simulink model "Model_Predictive_Controller"  (R2018a)
settings: Solver=VariableStepAuto  StartTime=0.0  StopTime=10.0  RelTol=1e-3
libraries: Meldas_library x2, mpclib x1
settings Model: Creator=KAARTIK  LastModifiedBy=KAARTIK

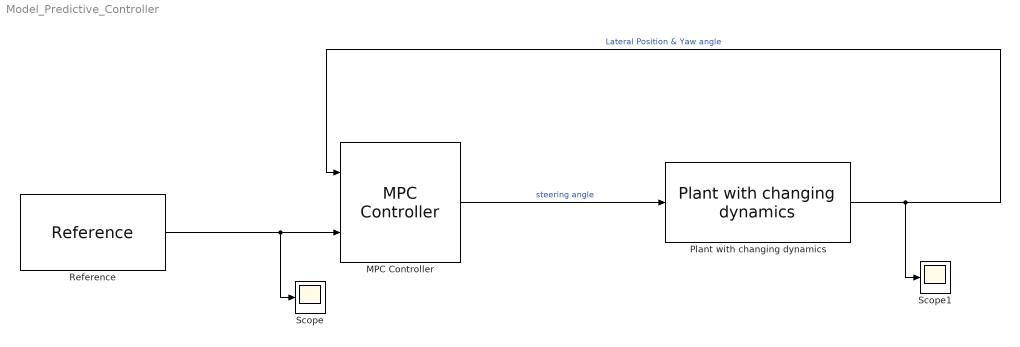
== system Model_Predictive_Controller ==
  MPC Controller : mpclib/MPC Controller  SCDEnableBlockLinearizationSpecification=on  is_multiple=0  enable_value=0  return_u0=off  updateMPCinCallerWorkspace=on  ref_from_ws=off  ref_signal_name=[]  ref_preview=off  md_from_ws=off  md_signal_name=[]  md_preview=off  from_project=off  project_file=MPCtask.mat  md_inport=off  mv_inport=off  cost_outport=off  return_sequence=off  return_qpstatus=off  return_state=off  state_inport=off  lims_inport=off  cc_inport=off  ywt_inport=off  is_designfromscratch=0  uwt_inport=off  duwt_inport=off  rhoeps_inport=off  uref_inport=off  n_ts=1  n_p=10  n_mv=1  n_md=1  n_ud=0  n_mo=1  n_uo=0  BlockDataType=double  SampleTimeInherited=off  switch_inport=off
  Plant with changing dynamics : Meldas_library/Plant with changing dynamics  Vx=15
  Reference : Meldas_library/Reference  SystemSampleTime=-1
  Scope : Scope
  Scope1 : Scope
  wires:
  MPC Controller/1 -> Plant with changing dynamics/1  "steering angle"
  Plant with changing dynamics/1 -> Scope1/1, MPC Controller/1  "Lateral Position & Yaw angle"
  Reference/1 -> Scope/1, MPC Controller/2
